simulink model "dvig_harness"  (R2023a)
settings: Solver=VariableStepAuto  StartTime=0.0  StopTime=10.0  RelTol=1e-3
libraries: SignalEditorBlockLib x1
settings Model: Creator=diontep  LastModifiedBy=diontep

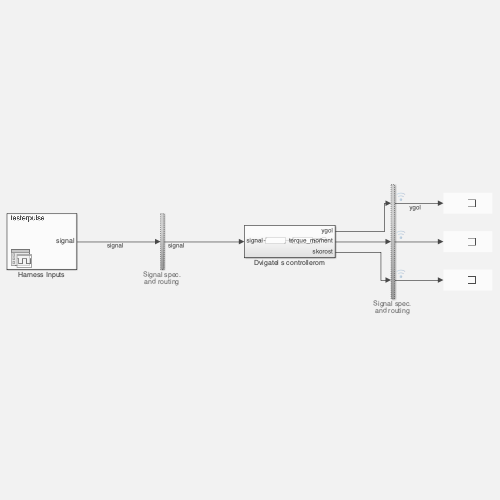
[thumbnail: Simulink's stored preview of the top-level diagram]
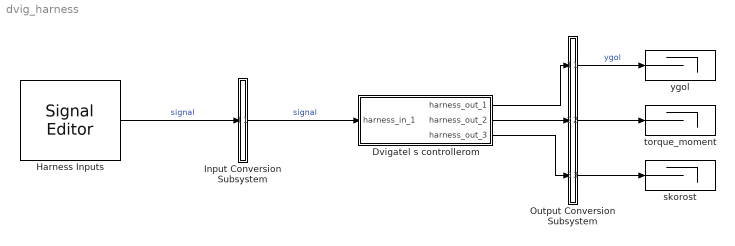
== system dvig_harness ==
  Dvigatel s controllerom : Subsystem  Tag=__SL_testing_harness_stub_
  Harness Inputs : SignalEditorBlockLib/Signal Editor  FileName=/Users/diontep/workspace/LR6/tests/dvig_harness_HarnessInputs.mat  ActiveScenario=testerpulse  ActiveSignal=signal  IsBus=off  OutputBusObjectStr=Bus: BusObject  SampleTime=0  Interpolate=off  ZeroCross=off  OutputAfterFinalValue=Setting to zero  Unit=inherit  PreserveSignalName=on  ApplySigPropsToAllScenarios=on
  Input Conversion Subsystem : Subsystem  Tag=__SLT_ICS__  Description=|
      | Signal spec.
      | and routing
      settings: AttributesFormatString=%<Description>
  Output Conversion Subsystem : Subsystem  Tag=__SLT_OCS__  Description=|
      | Signal spec.
      | and routing
      settings: AttributesFormatString=%<Description>
  skorost : Terminator
  torque_moment : Terminator
  ygol : Terminator
  wires:
  Harness Inputs/1 -> Input Conversion Subsystem/1(Inport_1)  "signal"
  Output Conversion Subsystem/1(Outport_1) -> ygol/1  "ygol"
  Output Conversion Subsystem/2(Outport_2) -> torque_moment/1
  Output Conversion Subsystem/3(Outport_3) -> skorost/1
  Input Conversion Subsystem/1(Outport_1) -> Dvigatel s controllerom/1(harness_in_1)  "signal"
  Dvigatel s controllerom/1(harness_out_1) -> Output Conversion Subsystem/1(Inport_1)
  Dvigatel s controllerom/2(harness_out_2) -> Output Conversion Subsystem/2(Inport_2)
  Dvigatel s controllerom/3(harness_out_3) -> Output Conversion Subsystem/3(Inport_3)

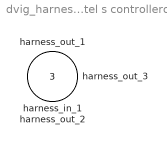
== system dvig_harness/Dvigatel s controllerom ==
  harness_in_1 : Inport
  harness_out_1 : Outport
  harness_out_2 : Outport  Port=2
  harness_out_3 : Outport  Port=3

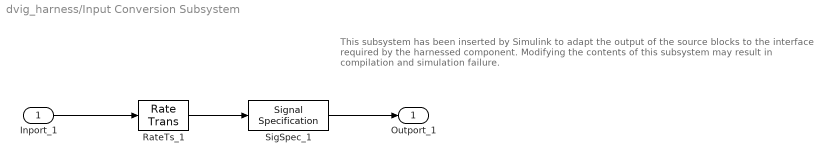
== system dvig_harness/Input Conversion Subsystem ==
  note: This subsystem has been inserted by Simulink to adapt the output of the source blocks to the interface required by the harnessed component.
      |  Modifying the contents of this subsystem may result in compilation and simulation failure.
  Inport_1 : Inport
  RateTs_1 : RateTransition  OutPortSampleTime=[-1, 0]
  SigSpec_1 : SignalSpecification  OutDataTypeStr=double  Dimensions=[1]  SampleTime=[-1, 0]
  Outport_1 : Outport
  wires:
  SigSpec_1/1 -> Outport_1/1
  RateTs_1/1 -> SigSpec_1/1
  Inport_1/1 -> RateTs_1/1

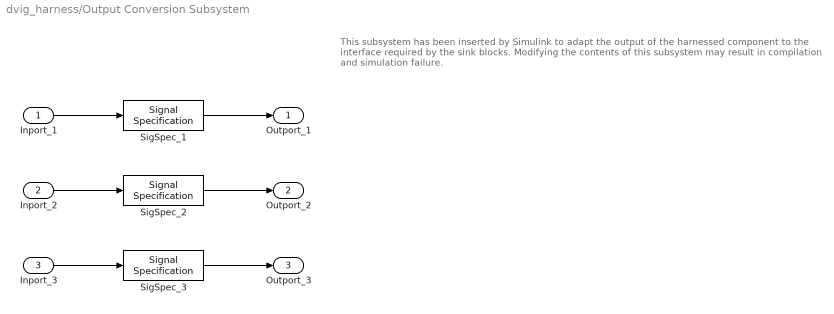
== system dvig_harness/Output Conversion Subsystem ==
  note: This subsystem has been inserted by Simulink to adapt the output of the harnessed component to the interface required by the sink blocks.
      |  Modifying the contents of this subsystem may result in compilation and simulation failure.
  Inport_1 : Inport
  Inport_2 : Inport  Port=2
  Inport_3 : Inport  Port=3
  SigSpec_1 : SignalSpecification  OutDataTypeStr=double  Dimensions=[1]
  SigSpec_2 : SignalSpecification  OutDataTypeStr=double  Dimensions=[1]
  SigSpec_3 : SignalSpecification  OutDataTypeStr=double  Dimensions=[1]
  Outport_1 : Outport
  Outport_2 : Outport  Port=2
  Outport_3 : Outport  Port=3
  wires:
  Inport_1/1 -> SigSpec_1/1
  SigSpec_1/1 -> Outport_1/1
  Inport_2/1 -> SigSpec_2/1
  SigSpec_2/1 -> Outport_2/1
  Inport_3/1 -> SigSpec_3/1
  SigSpec_3/1 -> Outport_3/1
